simulink model "sampleModel189"  (R2021b)
settings: Solver=VariableStepAuto  StartTime=0.0  StopTime=10.0  RelTol=1e-3
undefined symbols (not defined in the file or in its folder): magnitude, Newton, Raphson
libraries: simulink x11, slpidlib x1
settings Model: Creator=user  LastModifiedBy=user

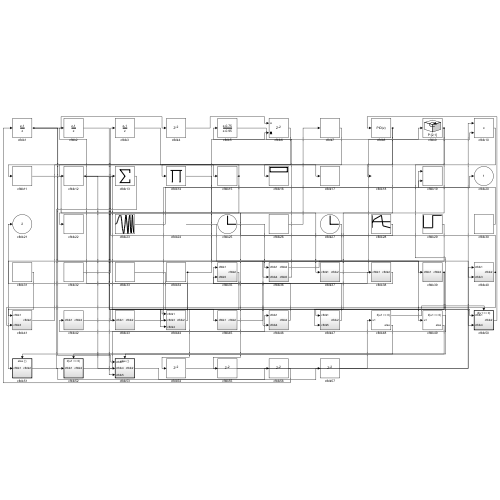
[thumbnail: Simulink's stored preview of the top-level diagram]
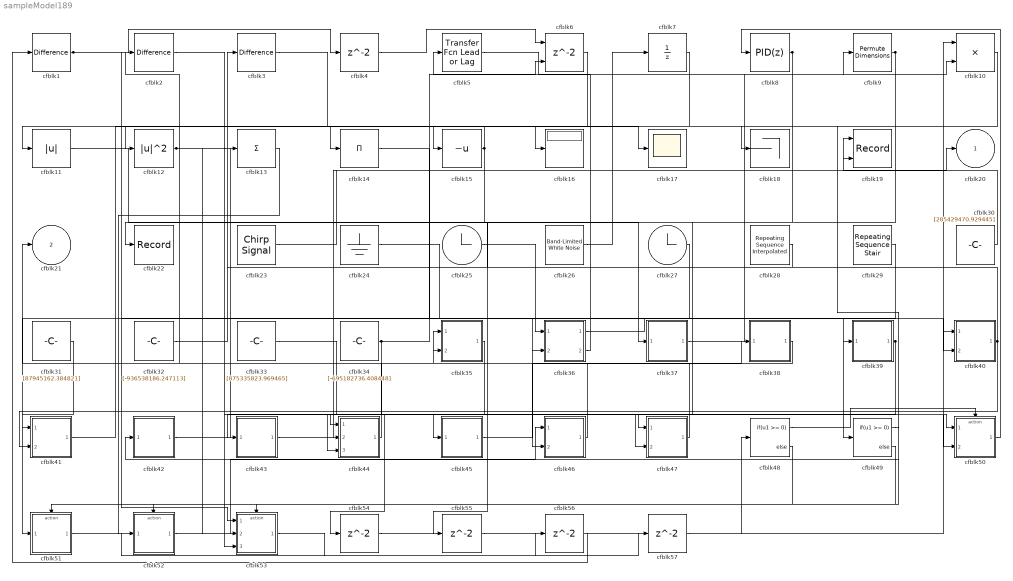
== system sampleModel189 ==
  cfblk1 : simulink/Discrete/Difference  ICPrevInput=0.0  OutMin=[]  OutMax=[]  OutDataTypeStr=Inherit: Inherit via back propagation  OutDataType=fixdt(1, 16)  OutScaling=2^-10  DoSatur=off
  cfblk10 : Product
  cfblk11 : Abs
  cfblk12 : Math  Operator=magnitude^2  SaturateOnIntegerOverflow=on
  cfblk13 : Sum  Inputs=+
  cfblk14 : Product  Inputs=*
  cfblk15 : UnaryMinus
  cfblk16 : Display
  cfblk17 : Scope
  cfblk18 : Terminator
  cfblk19 : Record  FileSettingsInternal="{\"entries\":[{\"content\":{\"excelSettings\":{\"content\":{},\"type\":\"Streamout.ExcelSettings\"}},\"type\":\"Streamout.FileSettingStorage\",\"uuid\":\"751e4d99-45f8-40d9-b9e3-6c58bf4239d2\"}],\"packageUris\":[\"http://schema.mathworks.com/mf0/streamout_blocks/R2020a\"],\"version\":\"1.0\"}"  Layout=[1 1]  SignalsInternal="{\"entries\":[{\"content\":{\"signals\":[{\"content\":{\"blockPath\":[\"sampleModel189/cfblk19\"],\"channel\":[],\"dimensions\":[1],\"domain\":\"sampleModel189/cfblk19\",\"lineColor\":\"#a2142f\",\"plots\":[1],\"port\":1,\"sid\":[\"\"],\"signalID\":7095,\"signalName\":\"cfblk30\"},\"type\":\"RecordBlkView.Signal\",\"uuid\":\"2f15c82b-8551-407f-94ab-65c4b1ae4010\"},{\"content\":{\"blockPath\":[\"sampleModel189/cfblk19\"],\"channel\":[],\"dimensions\":[1],\"domain\":\"sampleModel189/cfblk19\",\"lineColor\":\"#139fff\",\"plots\":[1],\"port\":2,\"sid\":[\"\"],\"signalID\":7099,\"signalName\":\"cfblk23\"},\"type\":\"RecordBlkView.Signal\",\"uuid\":\"093d831b-4d71-428b-aeeb-9270b93a471b\"}]},\"type\":\"RecordBlkView.InputSignals\",\"uuid\":\"52b7a778-21df-46cd-8200-b2327064ea82\"}],\"packageUris\":[\"http://schema.mathworks.com/mf0/streamout_blocks/R2020a\"],\"version\":\"1.0\"}"  VisualizationBindings="{\"xyplotplugin\":{\"info\":[{\"series\":[{\"bindingParametersList\":[{\"parameter\":\"X-Axis\",\"signalID\":7095,\"signalName\":\"cfblk30\"},{\"parameter\":\"Y-Axis\",\"signalID\":7099,\"signalName\":\"cfblk23\"}],\"seriesID\":10630}],\"subplotID\":1}]}}"  CompatibilityTag=XY
  cfblk2 : simulink/Discrete/Difference  ICPrevInput=0.0  OutMin=[]  OutMax=[]  OutDataTypeStr=Inherit: Inherit via back propagation  OutDataType=fixdt(1, 16)  OutScaling=2^-10  DoSatur=off
  cfblk22 : Record  FileSettingsInternal="{\"entries\":[{\"content\":{\"excelSettings\":{\"content\":{},\"type\":\"Streamout.ExcelSettings\"}},\"type\":\"Streamout.FileSettingStorage\",\"uuid\":\"a7b27562-a01f-4c86-8193-aa076a536ee6\"}],\"packageUris\":[\"http://schema.mathworks.com/mf0/streamout_blocks/R2020a\"],\"version\":\"1.0\"}"  SignalsInternal="{\"entries\":[{\"content\":{\"signals\":[{\"content\":{\"blockPath\":[\"sampleModel189/cfblk22\"],\"channel\":[],\"dimensions\":[1],\"domain\":\"sampleModel189/cfblk22\",\"lineColor\":\"#0072bd\",\"plots\":[1],\"port\":1,\"sid\":[\"\"],\"signalID\":7103,\"signalName\":\"cfblk28\"},\"type\":\"RecordBlkView.Signal\",\"uuid\":\"4461f903-eca4-4961-b801-cb7c5602d0fa\"}]},\"type\":\"RecordBlkView.InputSignals\",\"uuid\":\"5c4d19d6-a334-4d05-b301-3a9efca48321\"}],\"packageUris\":[\"http://schema.mathworks.com/mf0/streamout_blocks/R2020a\"],\"version\":\"1.0\"}"  VisualizationBindings="{\"sparklinesplugin\":{\"info\":[{\"bindingParametersList\":[],\"subplotID\":1}]}}"
  cfblk23 : simulink/Sources/Chirp Signal  f1=[936592796.660748]  T=[796240884.383840]  f2=[-728676324.872112]
  cfblk24 : Ground
  cfblk25 : Clock
  cfblk26 : simulink/Sources/Band-Limited White Noise  Cov=[1801458944.875940]  Ts=0.1  seed=[1962982381.000000]
  cfblk27 : Clock
  cfblk28 : simulink/Sources/Repeating Sequence Interpolated  OutValues=[-163031290.043030, 260540658.175411, 746721641.764119, -504290470.485012, -703877546.494160]  TimeValues=[0 0.1 0.5 0.6 1].'  LookUpMeth=Interpolation-Use End Values  tsamp=0.01  OutMin=[]  OutMax=[]  OutDataTypeStr=double  OutputDataTypeScalingMode=double  OutDataType=fixdt(0,8)  OutScaling=2^-10
  cfblk29 : simulink/Sources/Repeating Sequence Stair  OutValues=[-680152516.089759, -474003921.676535]  tsamp=-1  OutMin=[]  OutMax=[]  OutDataTypeStr=double  OutputDataTypeScalingMode=double  OutDataType=fixdt(0,8)  ConRadixGroup=Best Precision: Vector-wise  OutScaling=2^-12
  cfblk3 : simulink/Discrete/Difference  ICPrevInput=0.0  OutMin=[]  OutMax=[]  OutDataTypeStr=Inherit: Inherit via back propagation  OutDataType=fixdt(1, 16)  OutScaling=2^-10  DoSatur=off
  cfblk30 : Constant  Value=[285429470.929445]  SampleTime=1
  cfblk31 : Constant  Value=[87945162.384821]  SampleTime=1
  cfblk32 : Constant  Value=[-936538186.247113]  SampleTime=1
  cfblk33 : Constant  Value=[875335823.969465]  SampleTime=1
  cfblk34 : Constant  Value=[-695182736.408448]  SampleTime=1
  cfblk35 : Subsystem
  cfblk36 : Subsystem
  cfblk37 : Subsystem
  cfblk38 : Subsystem
  cfblk39 : Subsystem
  cfblk{4,54..57} (5 alike) : Delay  SampleTime=1
  cfblk40 : Subsystem
  cfblk41 : Subsystem
  cfblk42 : Subsystem
  cfblk43 : Subsystem
  cfblk44 : Subsystem
  cfblk45 : Subsystem
  cfblk46 : Subsystem
  cfblk47 : Subsystem
  cfblk48 : If  IfExpression=u1 >= 0  SampleTime=1
  cfblk49 : If  IfExpression=u1 >= 0  SampleTime=1
  cfblk5 : simulink/Discrete/Transfer Fcn Lead or Lag  PoleZ=0.95  ZeroZ=0.75  ICPrevOutput=0.0  ICPrevInput=0.0  DoSatur=off
      settings: SourceProductBaseCode=SL
  cfblk50 : Subsystem  TreatAsAtomicUnit=on
  cfblk51 : Subsystem  TreatAsAtomicUnit=on
  cfblk52 : Subsystem  TreatAsAtomicUnit=on
  cfblk53 : Subsystem  TreatAsAtomicUnit=on
  cfblk6 : Delay  ShowEnablePort=on  SampleTime=1
      settings: InputPortMap=u0,e6
  cfblk7 : UnitDelay  HasFrameUpgradeWarning=on
  cfblk8 : slpidlib/PID Controller  Controller=PID  Form=Parallel  TimeDomain=Discrete-time  UseExternalTs=off  SampleTime=1  IntegratorMethod=Forward Euler  FilterMethod=Forward Euler  ControllerParametersSource=internal  P=1  I=1  D=0  UseFilter=on  N=100  TunerSelectOption=Transfer Function Based (PID Tuner App)  InitialConditionSource=internal  InitialConditionForIntegrator=0  InitialConditionForFilter=0  DifferentiatorICPrevScaledInput=0  ExternalReset=none  TrackingMode=off  Kt=1  LimitOutput=off  SatLimitsSource=internal  UpperSaturationLimit=inf  LowerSaturationLimit=-inf  LinearizeAsGain=off  AntiWindupMode=none  Kb=1  POutMin=[]  POutMax=[]  IOutMin=[]  IOutMax=[]  DOutMin=[]  DOutMax=[]  NOutMin=[]  NOutMax=[]  SumOutMin=[]  SumOutMax=[]  SaturationOutMin=[]  SaturationOutMax=[]  PParamMin=[]  PParamMax=[]  IParamMin=[]  IParamMax=[]  DParamMin=[]  DParamMax=[]  NParamMin=[]  NParamMax=[]  KbParamMin=[]  KbParamMax=[]  KtParamMin=[]  KtParamMax=[]  KbOutMin=[]  KbOutMax=[]  KtOutMin=[]  KtOutMax=[]  IntegratorOutMin=[]  IntegratorOutMax=[]  FilterOutMin=[]  FilterOutMax=[]  SumI1OutMin=[]  SumI1OutMax=[]  SumI2OutMin=[]  SumI2OutMax=[]  SumI3OutMin=[]  SumI3OutMax=[]  SumI4OutMin=[]  SumI4OutMax=[]  SumDOutMin=[]  SumDOutMax=[]  DifferentiatorOutMin=[]  DifferentiatorOutMax=[]  FilterDiffOutCoefMin=[]  FilterDiffOutCoefMax=[]  ReciprocalOutMin=[]  ReciprocalOutMax=[]  SumDenOutMin=[]  SumDenOutMax=[]  SumNumOutMin=[]  SumNumOutMax=[]  DivideOutMin=[]  DivideOutMax=[]  UdiffTsProdOutMin=[]  UdiffTsProdOutMax=[]  NTsProdOutMin=[]  NTsProdOutMax=[]  UintegralTsProdOutMin=[]  UintegralTsProdOutMax=[]  UngainTsProdOutMin=[]  UngainTsProdOutMax=[]  IntegratorContinuousStateAttributes=''  IntegratorStateMustResolveToSignalObject=off  IntegratorRTWStateStorageClass=Auto  FilterContinuousStateAttributes=''  FilterStateMustResolveToSignalObject=off  FilterRTWStateStorageClass=Auto  ParallelPVariant=InternalParameters  IdealPVariant=Disabled  IVariant=InternalParameters  DVariant=InternalParameters  IntegratorVariant=Discrete  SatVariant=Disabled  AWVariant=Passthrough  PCopyVariant=Disabled  TRVariant=Disabled  FdbkBlocksVariant=Forward  IdealPFdbkVariant=Disabled  SatFdbkVariant=Disabled  DerivativeFilterVariant=ForwardEulerFilter  NVariant=InternalParameters  NCopyVariant=Disabled  FilterICVariant=InternalICsFilter  IntegratorICVariant=InternalICs  ExternalResetVariant=Disabled  TRSumVariant=Passthrough  SumFdbkVariant=Disabled  SumVariant=Sum_PID  TsampFilterVariant=InternalTs  TsampNgainVariant=Passthrough  TsampIntegralVariant=Passthrough  ExternalSaturationOutDataTypeStr=Inherit: Same as second input
  cfblk9 : PermuteDimensions
  cfblk20 : Outport
  cfblk21 : Outport  Port=2
  wires:
  cfblk24/1 -> cfblk49/1
  cfblk30/1 -> cfblk19/1
  cfblk26/1 -> cfblk7/1
  cfblk28/1 -> cfblk22/1
  cfblk13/1 -> cfblk52/1(cfblk1)
  cfblk9/1 -> cfblk42/1(cfblk1), cfblk47/1(cfblk1)
  cfblk41/1(cfblk2) -> cfblk15/1
  cfblk44/1(cfblk2) -> cfblk21/1
  cfblk43/1(cfblk2) -> cfblk20/1
  cfblk1/1 -> cfblk4/1, cfblk40/2(cfblk3), cfblk53/1(cfblk1)
  cfblk37/1(cfblk2) -> cfblk9/1
  cfblk8/1 -> cfblk18/1, cfblk55/1
  cfblk3/1 -> cfblk17/1
  cfblk42/1(cfblk2) -> cfblk45/1(cfblk1)
  cfblk47/1(cfblk2) -> cfblk2/1
  cfblk11/1 -> cfblk37/1(cfblk1)
  cfblk7/1 -> cfblk16/1
  cfblk52/1(cfblk2) -> cfblk46/1(cfblk1)
  cfblk6/1 -> cfblk14/1
  cfblk12/1 -> cfblk44/1(cfblk1), cfblk50/2(cfblk4), cfblk53/2(cfblk4)
  cfblk25/1 -> cfblk36/1(cfblk1)
  cfblk14/1 -> cfblk36/2(cfblk4)
  cfblk46/1(cfblk2) -> cfblk35/1(cfblk1)
  cfblk32/1 -> cfblk3/1
  cfblk27/1 -> cfblk46/2(cfblk4)
  cfblk50/1(cfblk2) -> cfblk8/1
  cfblk36/1(cfblk2) -> cfblk39/1(cfblk1)
  cfblk15/1 -> cfblk12/1, cfblk53/3(cfblk5)
  cfblk40/1(cfblk2) -> cfblk13/1, cfblk41/2(cfblk3)
  cfblk2/1 -> cfblk44/2(cfblk3)
  cfblk5/1 -> cfblk10/2
  cfblk34/1 -> cfblk43/1(cfblk1), cfblk6/2
  cfblk36/2(cfblk5) -> cfblk5/1
  cfblk39/1(cfblk2) -> cfblk44/3(cfblk4), cfblk47/2(cfblk5)
  cfblk23/1 -> cfblk19/2
  cfblk31/1 -> cfblk51/1(cfblk1)
  cfblk38/1(cfblk2) -> cfblk35/2(cfblk5)
  cfblk4/1 -> cfblk6/1
  cfblk33/1 -> cfblk50/1(cfblk1)
  cfblk29/1 -> cfblk41/1(cfblk1)
  cfblk45/1(cfblk2) -> cfblk38/1(cfblk1)
  cfblk10/1 -> cfblk11/1
  cfblk48/1 -> cfblk50/Action
  cfblk48/2 -> cfblk51/Action
  cfblk49/1 -> cfblk52/Action
  cfblk49/2 -> cfblk53/Action
  cfblk35/1(cfblk2) -> cfblk54/1
  cfblk54/1 -> cfblk10/1
  cfblk55/1 -> cfblk40/1(cfblk1)
  cfblk53/1(cfblk2) -> cfblk56/1
  cfblk56/1 -> cfblk1/1
  cfblk51/1(cfblk2) -> cfblk57/1
  cfblk57/1 -> cfblk48/1

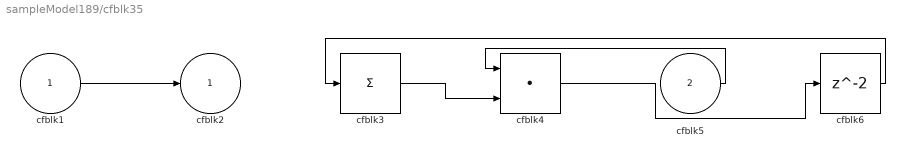
== system sampleModel189/cfblk35 ==
  cfblk1 : Inport
  cfblk5 : Inport  Port=2
  cfblk3 : Sum  Inputs=+
  cfblk4 : DotProduct  InputSameDT=on  OutDataTypeStr=Inherit: Inherit via internal rule
  cfblk6 : Delay  SampleTime=1
  cfblk2 : Outport
  wires:
  cfblk5/1 -> cfblk4/1
  cfblk1/1 -> cfblk2/1
  cfblk3/1 -> cfblk4/2
  cfblk4/1 -> cfblk6/1
  cfblk6/1 -> cfblk3/1

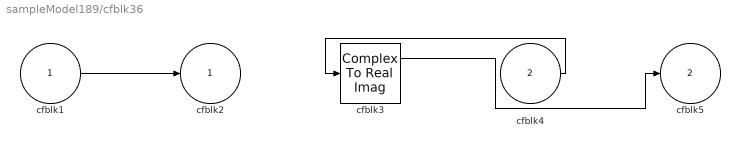
== system sampleModel189/cfblk36 ==
  cfblk1 : Inport
  cfblk4 : Inport  Port=2
  cfblk3 : ComplexToRealImag
  cfblk2 : Outport
  cfblk5 : Outport  Port=2
  wires:
  cfblk1/1 -> cfblk2/1
  cfblk4/1 -> cfblk3/1
  cfblk3/1 -> cfblk5/1

== system sampleModel189/cfblk37 ==
  cfblk1 : Inport
  cfblk3 : simulink/Discrete/Transfer Fcn Real Zero  ZeroZ=0.75  ICPrevInput=0.0  DoSatur=off
      settings: SourceProductBaseCode=SL
  cfblk2 : Outport
  wires:
  cfblk1/1 -> cfblk3/1
  cfblk3/1 -> cfblk2/1

== system sampleModel189/cfblk38 ==
  cfblk1 : Inport
  cfblk3 : Rounding
  cfblk2 : Outport
  wires:
  cfblk1/1 -> cfblk3/1
  cfblk3/1 -> cfblk2/1

== system sampleModel189/cfblk39 ==
  cfblk1 : Inport
  cfblk3 : PermuteDimensions
  cfblk2 : Outport
  wires:
  cfblk1/1 -> cfblk2/1, cfblk3/1

== system sampleModel189/cfblk40 ==
  cfblk1 : Inport
  cfblk3 : Inport  Port=2
  cfblk2 : Outport
  wires:
  cfblk3/1 -> cfblk2/1

== system sampleModel189/cfblk41 ==
  cfblk1 : Inport
  cfblk3 : Inport  Port=2
  cfblk2 : Outport
  wires:
  cfblk1/1 -> cfblk2/1

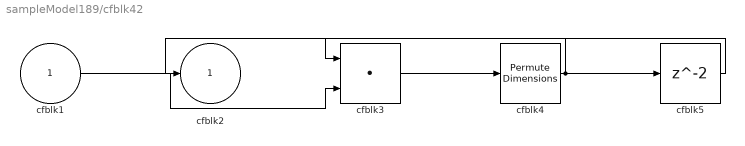
== system sampleModel189/cfblk42 ==
  cfblk1 : Inport
  cfblk3 : DotProduct  InputSameDT=on  OutDataTypeStr=Inherit: Inherit via internal rule
  cfblk4 : PermuteDimensions
  cfblk5 : Delay  SampleTime=1
  cfblk2 : Outport
  wires:
  cfblk4/1 -> cfblk2/1, cfblk5/1
  cfblk3/1 -> cfblk4/1
  cfblk1/1 -> cfblk3/2
  cfblk5/1 -> cfblk3/1

== system sampleModel189/cfblk43 ==
  cfblk1 : Inport
  cfblk3 : Gain  Gain=[-367020434.376307]
  cfblk2 : Outport
  wires:
  cfblk1/1 -> cfblk3/1
  cfblk3/1 -> cfblk2/1

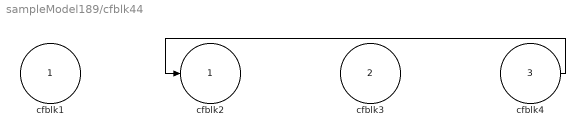
== system sampleModel189/cfblk44 ==
  cfblk1 : Inport
  cfblk3 : Inport  Port=2
  cfblk4 : Inport  Port=3
  cfblk2 : Outport
  wires:
  cfblk4/1 -> cfblk2/1

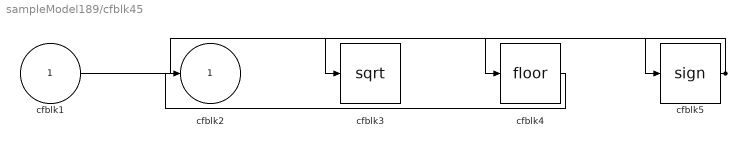
== system sampleModel189/cfblk45 ==
  cfblk1 : Inport
  cfblk3 : Sqrt  SaturateOnIntegerOverflow=on
  cfblk4 : Rounding
  cfblk5 : Signum
  cfblk2 : Outport
  wires:
  cfblk1/1 -> cfblk5/1
  cfblk4/1 -> cfblk2/1
  cfblk5/1 -> cfblk4/1, cfblk3/1

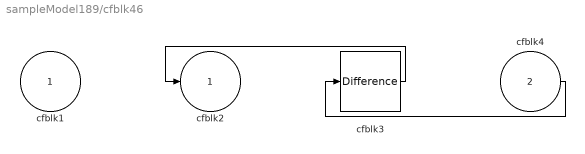
== system sampleModel189/cfblk46 ==
  cfblk1 : Inport
  cfblk4 : Inport  Port=2
  cfblk3 : simulink/Discrete/Difference  ICPrevInput=0.0  OutMin=[]  OutMax=[]  OutDataTypeStr=Inherit: Inherit via back propagation  OutDataType=fixdt(1, 16)  OutScaling=2^-10  DoSatur=off
  cfblk2 : Outport
  wires:
  cfblk3/1 -> cfblk2/1
  cfblk4/1 -> cfblk3/1

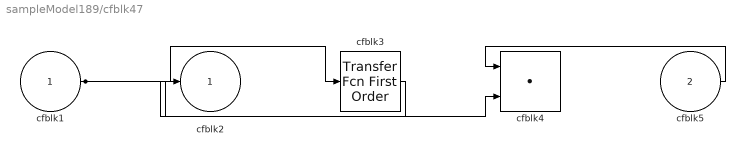
== system sampleModel189/cfblk47 ==
  cfblk1 : Inport
  cfblk5 : Inport  Port=2
  cfblk3 : simulink/Discrete/Transfer Fcn First Order  PoleZ=0.95  ICPrevOutput=0.0  DoSatur=off
  cfblk4 : DotProduct  InputSameDT=on  OutDataTypeStr=Inherit: Inherit via internal rule
  cfblk2 : Outport
  wires:
  cfblk1/1 -> cfblk3/1, cfblk4/2
  cfblk3/1 -> cfblk2/1
  cfblk5/1 -> cfblk4/1

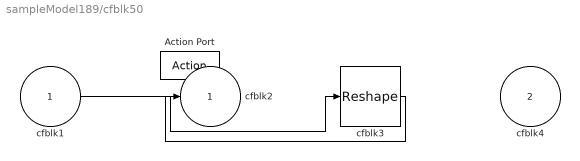
== system sampleModel189/cfblk50 ==
  cfblk1 : Inport
  cfblk4 : Inport  Port=2
  Action Port : ActionPort  ActionPortLabel=if(u1 >= 0)
  cfblk3 : Reshape
  cfblk2 : Outport
  wires:
  cfblk1/1 -> cfblk3/1
  cfblk3/1 -> cfblk2/1

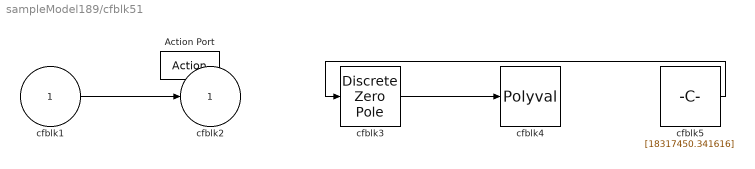
== system sampleModel189/cfblk51 ==
  cfblk1 : Inport
  Action Port : ActionPort  ActionPortLabel=else
  cfblk3 : DiscreteZeroPole  Poles=[0 0.5]  Gain=1  SampleTime=-1
  cfblk4 : Polyval  Coefs=[ +2.081618890e-019, -1.441693666e-014, +4.719686976e-010, -8.536869453e-006, +1.621573104e-001, -8.087801117e+001 ]
  cfblk5 : Constant  Value=[18317450.341616]  SampleTime=1
  cfblk2 : Outport
  wires:
  cfblk5/1 -> cfblk3/1
  cfblk3/1 -> cfblk4/1
  cfblk1/1 -> cfblk2/1

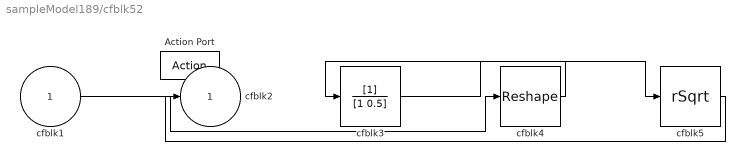
== system sampleModel189/cfblk52 ==
  cfblk1 : Inport
  Action Port : ActionPort  ActionPortLabel=if(u1 >= 0)
  cfblk3 : DiscreteFilter
  cfblk4 : Reshape
  cfblk5 : Sqrt  Operator=rSqrt  AlgorithmType=Newton-Raphson  SaturateOnIntegerOverflow=on
  cfblk2 : Outport
  wires:
  cfblk1/1 -> cfblk4/1
  cfblk4/1 -> cfblk3/1
  cfblk3/1 -> cfblk5/1
  cfblk5/1 -> cfblk2/1

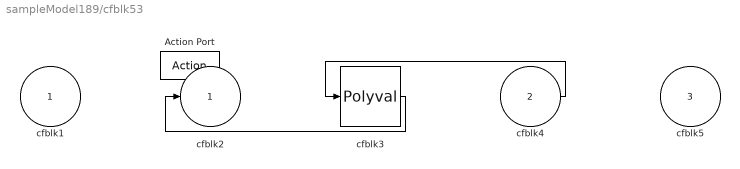
== system sampleModel189/cfblk53 ==
  cfblk1 : Inport
  cfblk4 : Inport  Port=2
  cfblk5 : Inport  Port=3
  Action Port : ActionPort  ActionPortLabel=else
  cfblk3 : Polyval  Coefs=[ +2.081618890e-019, -1.441693666e-014, +4.719686976e-010, -8.536869453e-006, +1.621573104e-001, -8.087801117e+001 ]
  cfblk2 : Outport
  wires:
  cfblk3/1 -> cfblk2/1
  cfblk4/1 -> cfblk3/1
